simulink model "maskedsaturation"  (R2022b)
settings: Solver=VariableStepAuto  StartTime=0.0  StopTime=10.0  RelTol=1e-3
settings Model: Creator=brbar  LastModifiedBy=brbar

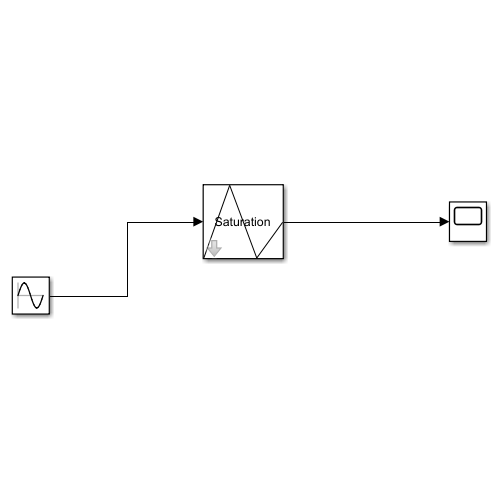
[thumbnail: Simulink's stored preview of the top-level diagram]
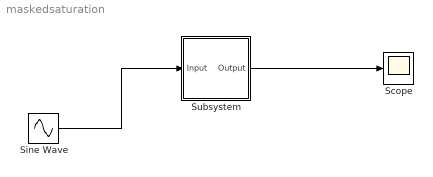
== system maskedsaturation ==
  Scope : Scope
  Sine Wave : Sin  Amplitude=10  SampleTime=0
  Subsystem : Subsystem  mask{upper=5, lower=-5}
      mask prompts: upper "Upper limit"; lower "Lower limit"
      mask DialogControl DescGroupVar Prompt: Saturation Block
      mask Display:
      | plot([10 20 30 40], [10 20 10 15]);
      | disp('Saturation');
  wires:
  Sine Wave/1 -> Subsystem/1(Input)
  Subsystem/1(Output) -> Scope/1

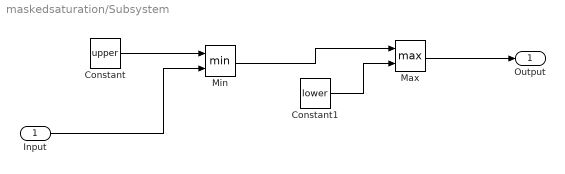
== system maskedsaturation/Subsystem ==
  Input : Inport
  Constant : Constant  Value=upper
  Constant1 : Constant  Value=lower
  Max : MinMax  Function=max  Inputs=2
  Min : MinMax  Inputs=2
  Output : Outport
  wires:
  Max/1 -> Output/1
  Min/1 -> Max/1
  Constant/1 -> Min/1
  Constant1/1 -> Max/2
  Input/1 -> Min/2
